simulink model "Tut8_RelationalOperator"  (R2021a)
settings: Solver=VariableStepAuto  StartTime=0.0  StopTime=10.0  RelTol=1e-3
settings Model: Creator=cheta  LastModifiedBy=cheta

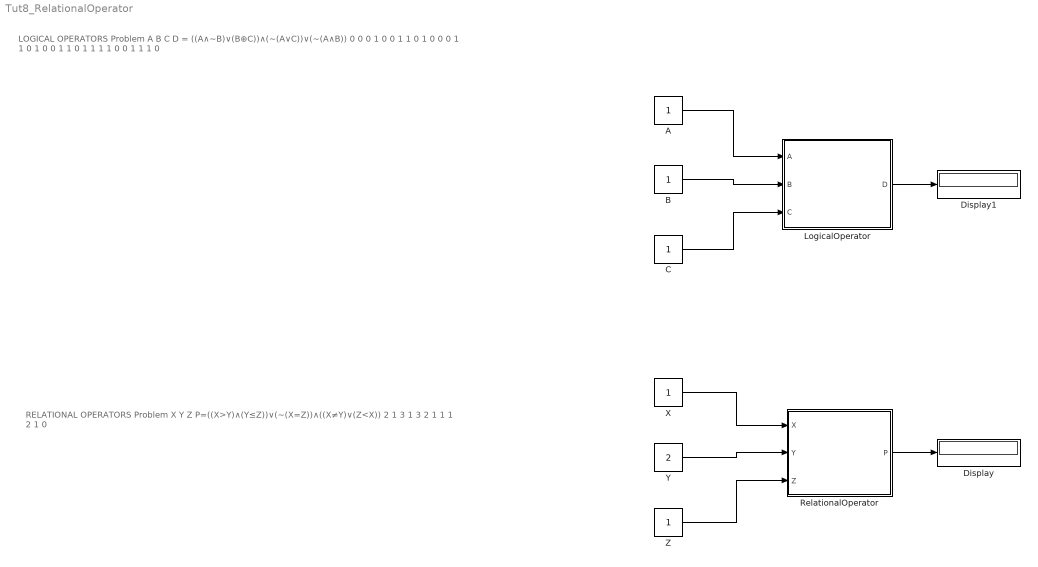
== system Tut8_RelationalOperator ==
  note: RELATIONAL OPERATORS Problem
      | X	Y	Z	            P=((X>Y)∧(Y≤Z))∨(∼(X=Z))∧((X≠Y)∨(Z<X))
      | 2	1	3	      	1
      | 3	2	1	       	1
      | 1	2	1			0
  note: LOGICAL OPERATORS Problem
      | A	B	C	                                    D = ((A∧∼B)∨(B⊕C))∧(∼(A∨C))∨(∼(A∧B))
      | 0	0	0	                                    1
      | 0	0	1	                                    1
      | 0	1	0	                                    0
      | 0	1	1	                                    0
      | 1	0	0	                                    1
      | 1	0	1	                                    1
      | 1	1	0	                                    0
      | 1	1	1	                                    0
  A : Constant
  B : Constant
  C : Constant
  Display : Display
  Display1 : Display
  LogicalOperator : Subsystem
  RelationalOperator : Subsystem
  X : Constant
  Y : Constant  Value=2
  Z : Constant
  wires:
  RelationalOperator/1(P) -> Display/1
  LogicalOperator/1(D) -> Display1/1
  A/1 -> LogicalOperator/1(A)
  B/1 -> LogicalOperator/2(B)
  C/1 -> LogicalOperator/3(C)
  X/1 -> RelationalOperator/1(X)
  Y/1 -> RelationalOperator/2(Y)
  Z/1 -> RelationalOperator/3(Z)

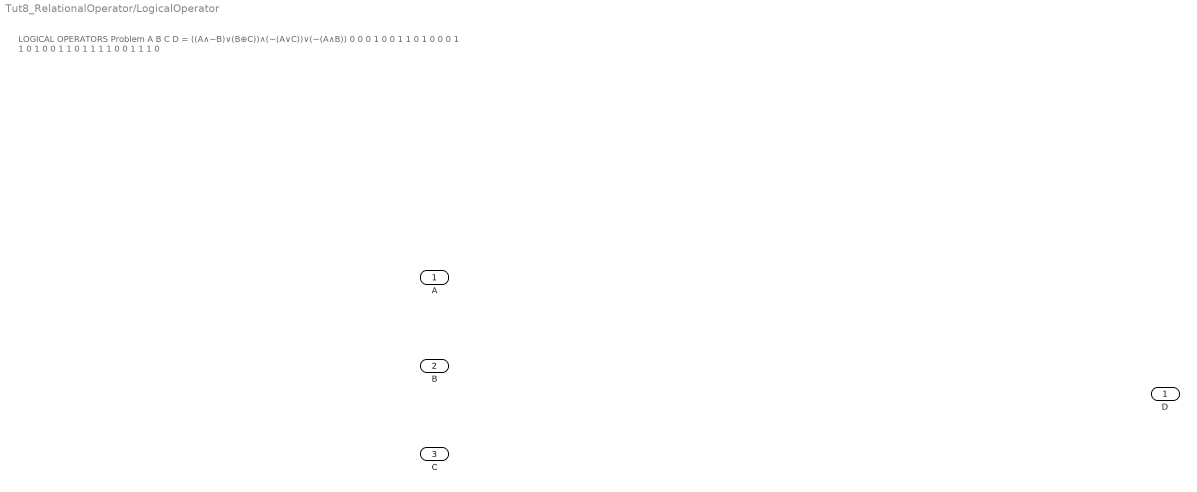
== system Tut8_RelationalOperator/LogicalOperator ==
  note: LOGICAL OPERATORS Problem
      | A	B	C	                                    D = ((A∧∼B)∨(B⊕C))∧(∼(A∨C))∨(∼(A∧B))
      | 0	0	0	                                    1
      | 0	0	1	                                    1
      | 0	1	0	                                    0
      | 0	1	1	                                    0
      | 1	0	0	                                    1
      | 1	0	1	                                    1
      | 1	1	0	                                    0
      | 1	1	1	                                    0
  A : Inport
  B : Inport  Port=2
  C : Inport  Port=3
  D : Outport

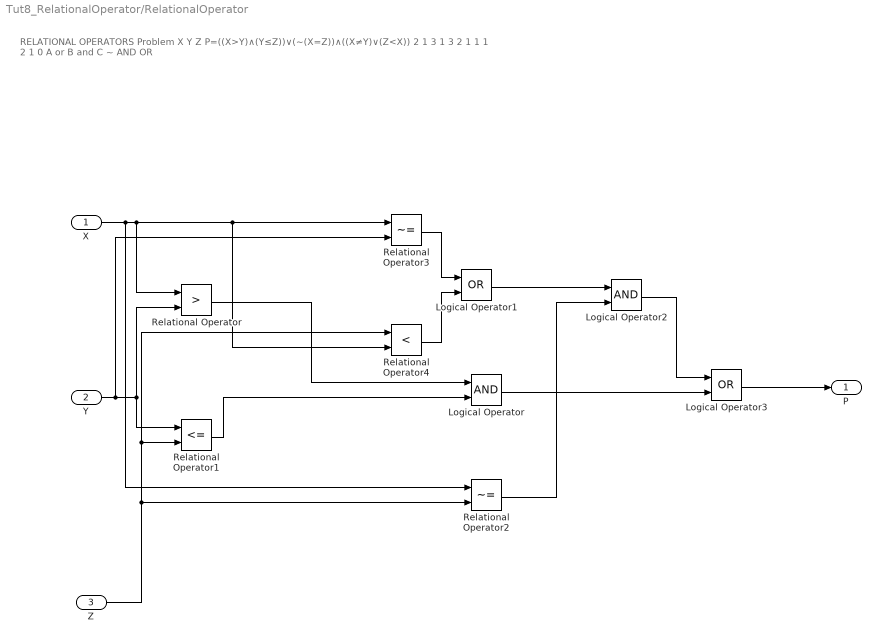
== system Tut8_RelationalOperator/RelationalOperator ==
  note: RELATIONAL OPERATORS Problem
      | X	Y	Z	            P=((X>Y)∧(Y≤Z))∨(∼(X=Z))∧((X≠Y)∨(Z<X))
      | 2	1	3	      	1
      | 3	2	1	       	1
      | 1	2	1			0
      | A or B and C
      | ~
      | AND
      | OR
  X : Inport
  Y : Inport  Port=2
  Z : Inport  Port=3
  Logical Operator : Logic  AllPortsSameDT=off  OutDataTypeStr=boolean
  Logical Operator1 : Logic  Operator=OR  AllPortsSameDT=off  OutDataTypeStr=boolean
  Logical Operator2 : Logic  AllPortsSameDT=off  OutDataTypeStr=boolean
  Logical Operator3 : Logic  Operator=OR  AllPortsSameDT=off  OutDataTypeStr=boolean
  Relational Operator : RelationalOperator  Operator=>  OutDataTypeStr=boolean  RndMeth=Simplest
  Relational Operator1 : RelationalOperator  Operator=<=  OutDataTypeStr=boolean  RndMeth=Simplest
  Relational Operator2 : RelationalOperator  Operator=~=  OutDataTypeStr=boolean  RndMeth=Simplest
  Relational Operator3 : RelationalOperator  Operator=~=  OutDataTypeStr=boolean  RndMeth=Simplest
  Relational Operator4 : RelationalOperator  Operator=<  OutDataTypeStr=boolean  RndMeth=Simplest
  P : Outport
  wires:
  X/1 -> Relational Operator2/1, Relational Operator4/2, Relational Operator3/1, Relational Operator/1
  Y/1 -> Relational Operator3/2, Relational Operator1/1, Relational Operator/2
  Z/1 -> Relational Operator4/1, Relational Operator1/2, Relational Operator2/2
  Relational Operator/1 -> Logical Operator/1
  Relational Operator1/1 -> Logical Operator/2
  Relational Operator3/1 -> Logical Operator1/1
  Relational Operator4/1 -> Logical Operator1/2
  Logical Operator1/1 -> Logical Operator2/1
  Relational Operator2/1 -> Logical Operator2/2
  Logical Operator2/1 -> Logical Operator3/1
  Logical Operator/1 -> Logical Operator3/2
  Logical Operator3/1 -> P/1
